simulink model "BallAndPlateSimulink"  (R2024b)
settings: Solver=VariableStepAuto  StartTime=0.0  StopTime=20  RelTol=1e-3
undefined symbols (not defined in the file or in its folder): Ad_p, Bd_p, Cd, DiscIntNeverNeededParam, Ki_d, Kp_d, Ld, Ts
settings Model: Creator=dacvo  LastModifiedBy=dacvo

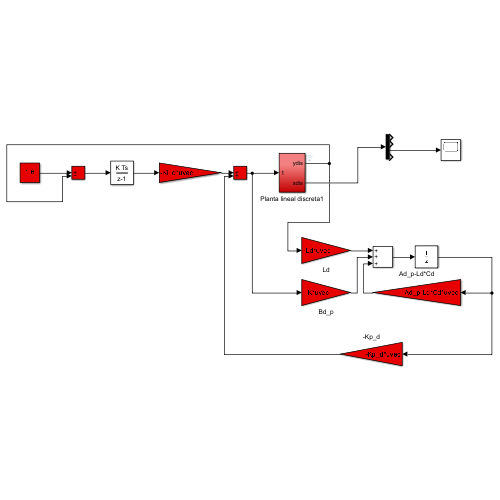
[thumbnail: Simulink's stored preview of the top-level diagram]
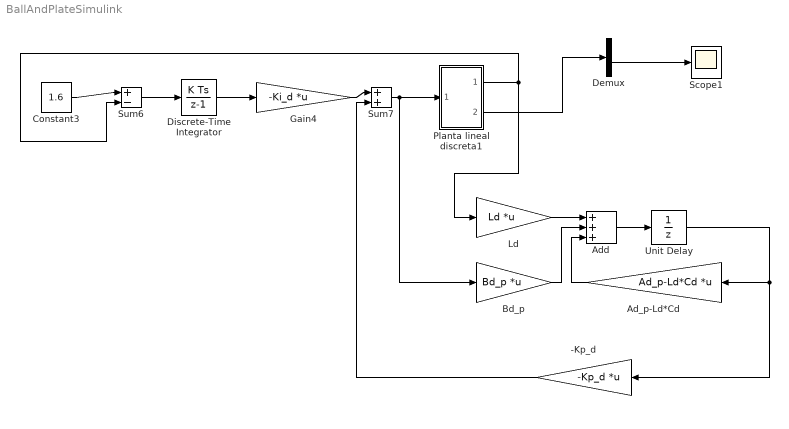
== system BallAndPlateSimulink ==
  -Kp_d : Gain  Gain=-Kp_d  Multiplication=Matrix(K*u) (u vector)  SampleTime=Ts
  Ad_p-Ld*Cd : Gain  Gain=Ad_p-Ld*Cd  Multiplication=Matrix(K*u) (u vector)  SampleTime=Ts
  Add : Sum  Inputs=+++
  Bd_p : Gain  Gain=Bd_p  Multiplication=Matrix(K*u) (u vector)  SampleTime=Ts
  Constant3 : Constant  Value=1.6  SampleTime=Ts
  Demux : Demux
  Discrete-Time Integrator : DiscreteIntegrator  SampleTime=Ts  ICPrevOutput=DiscIntNeverNeededParam  ICPrevScaledInput=DiscIntNeverNeededParam
  Gain4 : Gain  Gain=-Ki_d  Multiplication=Matrix(K*u) (u vector)  SampleTime=Ts
  Ld : Gain  Gain=Ld  Multiplication=Matrix(K*u) (u vector)  SampleTime=Ts
  Planta lineal discreta1 : Subsystem
  Scope1 : Scope
  Sum6 : Sum  Inputs=|+-
  Sum7 : Sum  Inputs=|++
  Unit Delay : UnitDelay  SampleTime=Ts  HasFrameUpgradeWarning=on
  wires:
  Constant3/1 -> Sum6/1
  Sum7/1 -> Bd_p/1, Planta lineal discreta1/1(In1)
  Gain4/1 -> Sum7/1
  Ld/1 -> Add/1
  Bd_p/1 -> Add/2
  Planta lineal discreta1/1(ydis) -> Ld/1, Sum6/2
  Discrete-Time Integrator/1 -> Gain4/1
  -Kp_d/1 -> Sum7/2
  Add/1 -> Unit Delay/1
  Ad_p-Ld*Cd/1 -> Add/3
  Unit Delay/1 -> -Kp_d/1, Ad_p-Ld*Cd/1
  Sum6/1 -> Discrete-Time Integrator/1
  Demux/3 -> Scope1/1
  Planta lineal discreta1/2(xdis) -> Demux/1

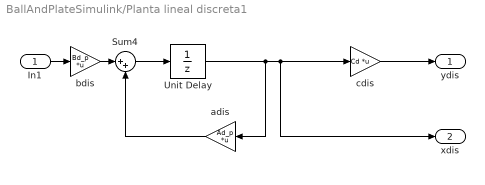
== system BallAndPlateSimulink/Planta lineal discreta1 ==
  In1 : Inport
  Sum4 : Sum  Inputs=|++
  Unit Delay : UnitDelay  SampleTime=Ts  HasFrameUpgradeWarning=on
  adis : Gain  Gain=Ad_p  Multiplication=Matrix(K*u) (u vector)  SampleTime=Ts
  bdis : Gain  Gain=Bd_p  Multiplication=Matrix(K*u) (u vector)  SampleTime=Ts
  cdis : Gain  Gain=Cd  Multiplication=Matrix(K*u) (u vector)  SampleTime=Ts
  ydis : Outport
  xdis : Outport  Port=2
  wires:
  bdis/1 -> Sum4/1
  Sum4/1 -> Unit Delay/1
  Unit Delay/1 -> adis/1, xdis/1, cdis/1
  adis/1 -> Sum4/2
  In1/1 -> bdis/1
  cdis/1 -> ydis/1
